simulink model "PSFB_topology_DCCharger"  (R2023a)
settings: Solver=ode23s  StartTime=0.0  StopTime=4  MaxStep=50e-6  RelTol=1e-4
undefined symbols (not defined in the file): Ion, Lithium
libraries: spsDiodeLib x10, spsCurrentMeasurementLib x4, spsMosfetLib x4, spsVoltageMeasurementLib x4, spsACVoltageSourceLib x3, spsSeriesRLCBranchLib x3, slpidlib x2, spspowerguiLib x2, spsBatteryLib x1, spsGroundLib x1, spsLinearTransformerLib x1, spsPowerLib x1
settings Model: Creator=zubin  LastModifiedBy=zubin

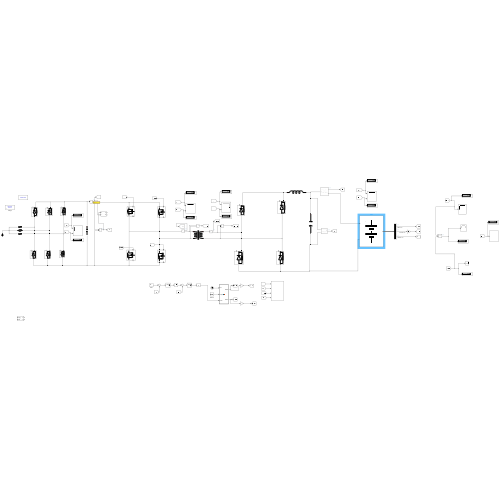
[thumbnail: Simulink's stored preview of the top-level diagram]
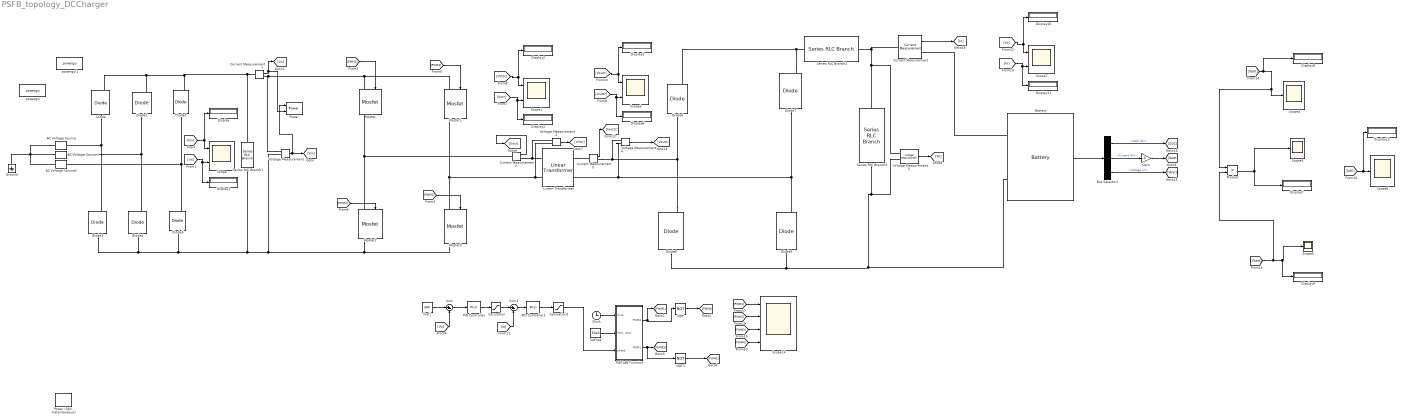
== system PSFB_topology_DCCharger ==
  AC Voltage Source : spsACVoltageSourceLib/AC Voltage Source  Amplitude=240  Phase=0  Frequency=50  SampleTime=0  Measurements=None  BusType=swing  Pref=30e3  Qref=10e3  Qmin=-inf  Qmax=+inf
  AC Voltage Source1 : spsACVoltageSourceLib/AC Voltage Source  Amplitude=240  Phase=-120  Frequency=50  SampleTime=0  Measurements=None  BusType=swing  Pref=30e3  Qref=10e3  Qmin=-inf  Qmax=+inf
  AC Voltage Source2 : spsACVoltageSourceLib/AC Voltage Source  Amplitude=230  Phase=120  Frequency=50  SampleTime=0  Measurements=None  BusType=swing  Pref=30e3  Qref=10e3  Qmin=-inf  Qmax=+inf
  Battery : spsBatteryLib/Battery  BatType=Lithium-Ion  ShowTempParam=off  ThermalPreset=no  ShowAgeParam=off  NomV=320  NomQ=94.5  SOC=80  Batt_Tr=5  PresetModel=on  MaxQ=94.5  MinV=240  FullV=372.4759  Dis_rate=41.087  R=0.033862  Normal_OP=85.4609  expZone="[345.7235      4.642826]"  current=[6.5 13 32.5]  Units=Time  Tci=20  NomT=20  T2=-30  MaxQ2=4.8  FullV2=7.1  Normal_OP2=5.655  expZone2="[6.58           1]"  Rca=0.6  ti=2000  Dp=0  Neq0=0  Tsim=1e6  Ta1=25  Qeol=5.4*0.9  Reol=0.013333*1.2  Char_age=[2.3478, 3]  Dis_age=[2.3478, 10]  N1=1500  N2=10500  N3=1000  N4=1400  Ta2=45  N5=950
      settings: LibrarySourceBlock=electricdrivelib/Extra Sources/Battery
  Bus Selector1 : BusSelector  OutputSignals=SOC (%),Current (A),Voltage (V)
  Clock : Clock
  Current Measurement{,1..3} (4 alike) : spsCurrentMeasurementLib/Current Measurement  PhasorSimulation=off  OutputType=Complex  PSBequivalent=0
  Diode{,1..9} (10 alike) : spsDiodeLib/Diode  Ron=0.001  Lon=0  Vf=0.8  IC=0  UseSnubber=0  Rs=500  Cs=250e-9  Measurements=on
  Display{,1..3,5..12} (12 alike) : Display
  Gain : Gain  Gain=-1
  Ground : spsGroundLib/Ground  LConnTagsString=a
  Linear Transformer : spsLinearTransformerLib/Linear Transformer  UNITS=SI  NominalPower=[ 100e3 50e3 ]  winding1=[415 9e-6 0.009e-6]  winding2=[360 4e-9 0.033e-9]  ThreeWindings=off  winding3=[3.15e+05 6.615 0.84225]  RmLm=[5.3445e6 28.66]  Measurements=None  DataType=on
  MATLAB Function : MATLAB Function  TreatAsAtomicUnit=on
  Mosfet{,1..3} (4 alike) : spsMosfetLib/Mosfet  Ron=0.1  Lon=0  Rd=0.01  Vfd=0  IC=0  Rs=1e5  Cs=inf  Measurements=on
  NOT : Logic  Operator=NOT  IconShape=distinctive  AllPortsSameDT=off  OutDataTypeStr=boolean
  NOT1 : Logic  Operator=NOT  IconShape=distinctive  AllPortsSameDT=off  OutDataTypeStr=boolean
  PID Controller : slpidlib/PID Controller  Controller=PI  Form=Parallel  TimeDomain=Continuous-time  UseExternalTs=off  SampleTime=-1  IntegratorMethod=Forward Euler  FilterMethod=Forward Euler  ControllerParametersSource=internal  P=50000  I=500000  UseKiTs=off  D=0  N=100  UseFilter=on  TunerSelectOption=Transfer Function Based (PID Tuner App)  InitialConditionSource=internal  InitialConditionForIntegrator=0  InitialConditionForFilter=0  DifferentiatorICPrevScaledInput=0  ExternalReset=none  TrackingMode=off  Kt=1  LimitOutput=on  SatLimitsSource=internal  UpperSaturationLimit=180  LowerSaturationLimit=-inf  LinearizeAsGain=on  AntiWindupMode=none  Kb=1  LimitIntegrator=off  UpperIntegratorSaturationLimit=inf  LowerIntegratorSaturationLimit=-inf  POutMin=[]  POutMax=[]  IOutMin=[]  IOutMax=[]  DOutMin=[]  DOutMax=[]  NOutMin=[]  NOutMax=[]  SumOutMin=[]  SumOutMax=[]  SaturationOutMin=[]  SaturationOutMax=[]  PParamMin=[]  PParamMax=[]  IParamMin=[]  IParamMax=[]  DParamMin=[]  DParamMax=[]  NParamMin=[]  NParamMax=[]  KbParamMin=[]  KbParamMax=[]  KtParamMin=[]  KtParamMax=[]  KbOutMin=[]  KbOutMax=[]  KtOutMin=[]  KtOutMax=[]  IntegratorOutMin=[]  IntegratorOutMax=[]  FilterOutMin=[]  FilterOutMax=[]  SumI1OutMin=[]  SumI1OutMax=[]  SumI2OutMin=[]  SumI2OutMax=[]  SumI3OutMin=[]  SumI3OutMax=[]  SumI4OutMin=[]  SumI4OutMax=[]  SumDOutMin=[]  SumDOutMax=[]  DifferentiatorOutMin=[]  DifferentiatorOutMax=[]  FilterDiffOutCoefMin=[]  FilterDiffOutCoefMax=[]  ReciprocalOutMin=[]  ReciprocalOutMax=[]  SumDenOutMin=[]  SumDenOutMax=[]  SumNumOutMin=[]  SumNumOutMax=[]  DivideOutMin=[]  DivideOutMax=[]  UdiffTsProdOutMin=[]  UdiffTsProdOutMax=[]  NTsProdOutMin=[]  NTsProdOutMax=[]  UintegralTsProdOutMin=[]  UintegralTsProdOutMax=[]  UngainTsProdOutMin=[]  UngainTsProdOutMax=[]  ClampingZeroOutDataTypeStr=Inherit: Inherit via back propagation  ClampingZeroOutMin=[]  ClampingZeroOutMax=[]  FilterDenConstantOutDataTypeStr=Inherit: Inherit via back propagation  FilterDenConstantOutMin=[]  FilterDenConstantOutMax=[]  PCopyOutDataTypeStr=Inherit: Inherit via back propagation  PCopyOutMin=[]  PCopyOutMax=[]  NCopyOutDataTypeStr=Inherit: Inherit via back propagation  NCopyOutMin=[]  NCopyOutMax=[]  IntegratorContinuousStateAttributes=''  IntegratorStateMustResolveToSignalObject=off  IntegratorRTWStateStorageClass=Auto  FilterContinuousStateAttributes=''  FilterStateMustResolveToSignalObject=off  FilterRTWStateStorageClass=Auto  ParallelPVariant=InternalParameters  IdealPVariant=Disabled  IVariant=InternalParameters  DVariant=Disabled  IntegratorVariant=Continuous  SatVariant=Enabled  AWVariant=Passthrough  PCopyVariant=Disabled  TRVariant=Disabled  FdbkBlocksVariant=Forward  IdealPFdbkVariant=Disabled  SatFdbkVariant=Disabled  DerivativeFilterVariant=Disabled  NVariant=Disabled  NCopyVariant=Disabled_SignalSpec  FilterICVariant=Disabled  IntegratorICVariant=InternalICs  ExternalResetVariant=Disabled  TRSumVariant=Passthrough  SumFdbkVariant=Disabled  SumVariant=Sum_PI  TsampFilterVariant=InternalTs  TsampNgainVariant=Passthrough  TsampIntegralVariant=Disabled_SignalSpec  ExternalSaturationOutDataTypeStr=Inherit: Same as second input
  PID Controller1 : slpidlib/PID Controller  Controller=PI  Form=Parallel  TimeDomain=Continuous-time  UseExternalTs=off  SampleTime=-1  IntegratorMethod=Forward Euler  FilterMethod=Forward Euler  ControllerParametersSource=internal  P=50000  I=50000  UseKiTs=off  D=0  N=100  UseFilter=on  TunerSelectOption=Transfer Function Based (PID Tuner App)  InitialConditionSource=internal  InitialConditionForIntegrator=0  InitialConditionForFilter=0  DifferentiatorICPrevScaledInput=0  ExternalReset=none  TrackingMode=off  Kt=1  LimitOutput=on  SatLimitsSource=internal  UpperSaturationLimit=180  LowerSaturationLimit=-inf  LinearizeAsGain=on  AntiWindupMode=none  Kb=1  LimitIntegrator=off  UpperIntegratorSaturationLimit=inf  LowerIntegratorSaturationLimit=-inf  POutMin=[]  POutMax=[]  IOutMin=[]  IOutMax=[]  DOutMin=[]  DOutMax=[]  NOutMin=[]  NOutMax=[]  SumOutMin=[]  SumOutMax=[]  SaturationOutMin=[]  SaturationOutMax=[]  PParamMin=[]  PParamMax=[]  IParamMin=[]  IParamMax=[]  DParamMin=[]  DParamMax=[]  NParamMin=[]  NParamMax=[]  KbParamMin=[]  KbParamMax=[]  KtParamMin=[]  KtParamMax=[]  KbOutMin=[]  KbOutMax=[]  KtOutMin=[]  KtOutMax=[]  IntegratorOutMin=[]  IntegratorOutMax=[]  FilterOutMin=[]  FilterOutMax=[]  SumI1OutMin=[]  SumI1OutMax=[]  SumI2OutMin=[]  SumI2OutMax=[]  SumI3OutMin=[]  SumI3OutMax=[]  SumI4OutMin=[]  SumI4OutMax=[]  SumDOutMin=[]  SumDOutMax=[]  DifferentiatorOutMin=[]  DifferentiatorOutMax=[]  FilterDiffOutCoefMin=[]  FilterDiffOutCoefMax=[]  ReciprocalOutMin=[]  ReciprocalOutMax=[]  SumDenOutMin=[]  SumDenOutMax=[]  SumNumOutMin=[]  SumNumOutMax=[]  DivideOutMin=[]  DivideOutMax=[]  UdiffTsProdOutMin=[]  UdiffTsProdOutMax=[]  NTsProdOutMin=[]  NTsProdOutMax=[]  UintegralTsProdOutMin=[]  UintegralTsProdOutMax=[]  UngainTsProdOutMin=[]  UngainTsProdOutMax=[]  ClampingZeroOutDataTypeStr=Inherit: Inherit via back propagation  ClampingZeroOutMin=[]  ClampingZeroOutMax=[]  FilterDenConstantOutDataTypeStr=Inherit: Inherit via back propagation  FilterDenConstantOutMin=[]  FilterDenConstantOutMax=[]  PCopyOutDataTypeStr=Inherit: Inherit via back propagation  PCopyOutMin=[]  PCopyOutMax=[]  NCopyOutDataTypeStr=Inherit: Inherit via back propagation  NCopyOutMin=[]  NCopyOutMax=[]  IntegratorContinuousStateAttributes=''  IntegratorStateMustResolveToSignalObject=off  IntegratorRTWStateStorageClass=Auto  FilterContinuousStateAttributes=''  FilterStateMustResolveToSignalObject=off  FilterRTWStateStorageClass=Auto  ParallelPVariant=InternalParameters  IdealPVariant=Disabled  IVariant=InternalParameters  DVariant=Disabled  IntegratorVariant=Continuous  SatVariant=Enabled  AWVariant=Passthrough  PCopyVariant=Disabled  TRVariant=Disabled  FdbkBlocksVariant=Forward  IdealPFdbkVariant=Disabled  SatFdbkVariant=Disabled  DerivativeFilterVariant=Disabled  NVariant=Disabled  NCopyVariant=Disabled_SignalSpec  FilterICVariant=Disabled  IntegratorICVariant=InternalICs  ExternalResetVariant=Disabled  TRSumVariant=Passthrough  SumFdbkVariant=Disabled  SumVariant=Sum_PI  TsampFilterVariant=InternalTs  TsampNgainVariant=Passthrough  TsampIntegralVariant=Disabled_SignalSpec  ExternalSaturationOutDataTypeStr=Inherit: Same as second input
  Power : spsPowerLib/Power  Freq=50  Vinit=[240, 0]  Iinit=[75, 0]  Ts=0
  "Power (3ph, Instantaneous)" : spsPower3phInstantaneousLib/Power (3ph, Instantaneous)
  Product : Product
  Saturation : Saturate  UpperLimit=100  LowerLimit=0
  Saturation1 : Saturate  UpperLimit=180  LowerLimit=0
  Scope{,1..2,7} (4 alike) : Scope  NumInputPorts=2
  Scope14 : Scope  NumInputPorts=4
  Scope{4..6,9} (4 alike) : Scope
  Series RLC Branch1 : spsSeriesRLCBranchLib/Series RLC Branch  LConnTagsString=__new0  RConnTagsString=__new0  BranchType=C  Resistance=1  Inductance=1e-3  SetiL0=off  InitialCurrent=0  Capacitance=500e-3  Setx0=off  InitialVoltage=0  Measurements=None
  Series RLC Branch2 : spsSeriesRLCBranchLib/Series RLC Branch  LConnTagsString=__new0  RConnTagsString=__new0  BranchType=L  Resistance=1  Inductance=0.08275e-6  SetiL0=off  InitialCurrent=0  Capacitance=33.6e-6  Setx0=off  InitialVoltage=0  Measurements=None
  Series RLC Branch3 : spsSeriesRLCBranchLib/Series RLC Branch  LConnTagsString=__new0  RConnTagsString=__new0  BranchType=C  Resistance=1  Inductance=3.9502e-5  SetiL0=off  InitialCurrent=0  Capacitance=484.17e-5  Setx0=off  InitialVoltage=0  Measurements=None
  Sum : Sum  Inputs=|+-
  Sum1 : Sum  Inputs=|+-
  SwFreq : Constant  Value=50e3
  Voltage Measurement{,2,4..5} (4 alike) : spsVoltageMeasurementLib/Voltage Measurement  PhasorSimulation=off  OutputType=Complex  PSBequivalent=0
  Vref1 : Constant  Value=360
  powergui : spspowerguiLib/powergui  Priority=1  SimulationMode=Discrete  SampleTime=1e-6  frequency=60  Iterations=50  frequencyindice=50  Pbase=100e6  ErrMax=1e-4  UnitsV=kV  UnitsW=MW  buscounter=0  FunctionMessages=off  echomessages=off  EnableUseOfTLC=off  CurrentSourceSwitches=off  DisableSnubberDevices=off  DisableRonSwitches=off  DisableVfSwitches=off  DisplayEquations=off  AutomaticDiscreteSolvers=off  SolverType=Tustin/Backward Euler (TBE)  Interpol=off  ExternalGateDelay=off  methode=off  Ts=100  x0status=blocks  SPID=on  SwTol=0  HookPort=off  NonlinearTolerance=1e-4  nMaxIteration=100  ContinueOnMaxIteration=off  RestoreLinks=warning  ResistiveCurrentMeasurement=off  Frange=[0:2:500]  Ylog=off  Xlog=on  ShowGrid=off  save=off  variable=ZData  structure=0  ZoomFFT=off  StartTime=0.0  cycles=1  DisplayStyle=1  fundamental=60  FreqAxis=off  MaxFrequency=1000  frequencyindicesteady=1  RmsSteady=1  display=off
  powergui1 : spspowerguiLib/powergui  Priority=1  SimulationMode=Continuous  SampleTime=1e-6  frequency=60  Iterations=50  frequencyindice=50  Pbase=100e6  ErrMax=1e-4  UnitsV=kV  UnitsW=MW  buscounter=0  FunctionMessages=off  echomessages=off  EnableUseOfTLC=off  CurrentSourceSwitches=off  DisableSnubberDevices=off  DisableRonSwitches=off  DisableVfSwitches=off  DisplayEquations=off  AutomaticDiscreteSolvers=off  SolverType=Tustin/Backward Euler (TBE)  Interpol=off  ExternalGateDelay=off  methode=off  Ts=100  x0status=blocks  SPID=on  SwTol=0  HookPort=off  NonlinearTolerance=1e-4  nMaxIteration=100  ContinueOnMaxIteration=off  RestoreLinks=warning  ResistiveCurrentMeasurement=off  Frange=[0:2:500]  Ylog=off  Xlog=on  ShowGrid=off  save=off  variable=ZData  structure=0  ZoomFFT=off  StartTime=0.0  cycles=1  DisplayStyle=1  fundamental=60  FreqAxis=off  MaxFrequency=1000  frequencyindicesteady=1  RmsSteady=1  display=off
  wires:
  Saturation1/1 -> MATLAB Function/3(phase)
  Voltage Measurement5/1 -> [Vo]
  Sum1/1 -> PID Controller1/1
  Bus Selector1/3 -> [Vbatt]  "<Voltage (V)>"
  Saturation/1 -> Sum1/1
  Voltage Measurement/1 -> Power/1, [Vin]
  Clock/1 -> MATLAB Function/1(time)
  [PWM2] -> Scope14/2
  PID Controller/1 -> Saturation/1
  [PWM4] -> Scope14/4
  [PWM3] -> Scope14/3
  [Iouttr] -> Display6/1, Scope2/2
  [PWM1] -> Scope14/1
  Current Measurement3/1 -> [Iouttr]
  [PWM4] -> Mosfet2/1
  NOT1/1 -> [PWM2]
  [PWM3] -> Mosfet1/1
  [Io] -> Display11/1, Scope7/2
  Vref1/1 -> Sum/1
  [Iin] -> Display1/1, Scope/2
  [IIntr] -> Display3/1, Scope1/2
  MATLAB Function/1(PWM2) -> [PWM1], NOT/1
  Current Measurement1/1 -> Power/2, [Iin]
  [Vin] -> Display/1, Scope/1
  [VIntr] -> Display2/1, Scope1/1
  Sum/1 -> PID Controller/1
  [PWM2] -> Mosfet3/1
  PID Controller1/1 -> Saturation1/1
  Voltage Measurement4/1 -> [Voutr]
  Current Measurement2/1 -> [IIntr]
  Bus Selector1/1 -> [SOC]  "<SOC (%)>"
  Bus Selector1/2 -> Gain/1  "<Current (A)>"
  Battery/1 -> Bus Selector1/1
  [PWM1] -> Mosfet/1
  [Vo] -> Display10/1, Scope7/1
  SwFreq/1 -> MATLAB Function/2(frequency)
  [Vo] -> Sum/2
  [Ibatt] -> Display8/1, Product/1, Scope4/1
  Current Measurement/1 -> [Io]
  [SOC] -> Display12/1, Scope6/1
  Product/1 -> Display7/1, Scope9/1
  [Vbatt] -> Product/2, Display9/1, Scope5/1
  [Voutr] -> Display5/1, Scope2/1
  Voltage Measurement2/1 -> [VIntr]
  Gain/1 -> [Ibatt]
  [Io] -> Sum1/2
  NOT/1 -> [PWM4]
  MATLAB Function/2(PWM1) -> NOT1/1, [PWM3]
  connections:
  Mosfet/RConn1 -- Mosfet2/LConn1 -- Current Measurement2/LConn1
  Linear Transformer/RConn2 -- Diode9/RConn1 -- Diode7/LConn1 -- Voltage Measurement4/LConn2
  Diode2/LConn1 -- Diode5/RConn1 -- AC Voltage Source2/RConn1
  Mosfet3/LConn1 -- Linear Transformer/LConn2 -- Voltage Measurement2/LConn2 -- Mosfet1/RConn1
  Current Measurement1/LConn1 -- Diode/RConn1 -- Diode1/RConn1 -- Diode2/RConn1 -- Series RLC Branch1/LConn1
  Voltage Measurement5/LConn1 -- Series RLC Branch3/LConn1 -- Series RLC Branch2/RConn1 -- Current Measurement/LConn1
  Linear Transformer/LConn1 -- Current Measurement2/RConn1 -- Voltage Measurement2/LConn1
  AC Voltage Source/LConn1 -- Ground/LConn1 -- AC Voltage Source1/LConn1 -- AC Voltage Source2/LConn1
  Diode/LConn1 -- Diode3/RConn1 -- AC Voltage Source/RConn1
  AC Voltage Source1/RConn1 -- Diode1/LConn1 -- Diode4/RConn1
  Diode5/LConn1 -- Mosfet3/RConn1 -- Mosfet2/RConn1 -- Voltage Measurement/LConn2 -- Series RLC Branch1/RConn1 -- Diode3/LConn1 -- Diode4/LConn1
  Diode9/LConn1 -- Diode8/LConn1 -- Series RLC Branch3/RConn1 -- Voltage Measurement5/LConn2 -- Battery/LConn2
  Diode7/RConn1 -- Series RLC Branch2/LConn1 -- Diode6/RConn1
  Voltage Measurement/LConn1 -- Current Measurement1/RConn1 -- Mosfet/LConn1 -- Mosfet1/LConn1
  Diode8/RConn1 -- Current Measurement3/RConn1 -- Voltage Measurement4/LConn1 -- Diode6/LConn1
  Linear Transformer/RConn1 -- Current Measurement3/LConn1
  Battery/LConn1 -- Current Measurement/RConn1

== matlab function PSFB_topology_DCCharger/MATLAB Function ==
  data: time input; PWM2 output; frequency input; phase input; PWM1 output
function [PWM2, PWM1] = fcn(time, frequency, phase) 
T_switching = 1/frequency; 
PWM1 = 0; PWM2 = 0; 
x = mod(time,T_switching); 
if x< T_switching/2 
    PWM1 = 1; 
end 
t_phi = T_switching*phase/360; 
y = mod(time+t_phi, T_switching); 
if y < T_switching/2 
    PWM2 = 1; 
end
